simulink model "engv2_Simscape_test_no_graphs"  (R2016a)
settings: Solver=ode23t  StartTime=0.0  StopTime=5790*3  MaxStep=0.1  RelTol=1e-6
libraries: fl_lib x26, nesl_utility x23, elec_lib x8, simulink x3
settings Model: Creator=Bruno  LastModifiedBy=Bruno
settings SolverCC: MaxConsecutiveZCs=10000  ZeroCrossAlgorithm=Adaptive  AlgebraicLoopSolver=LineSearch  SolverResetMethod=Robust

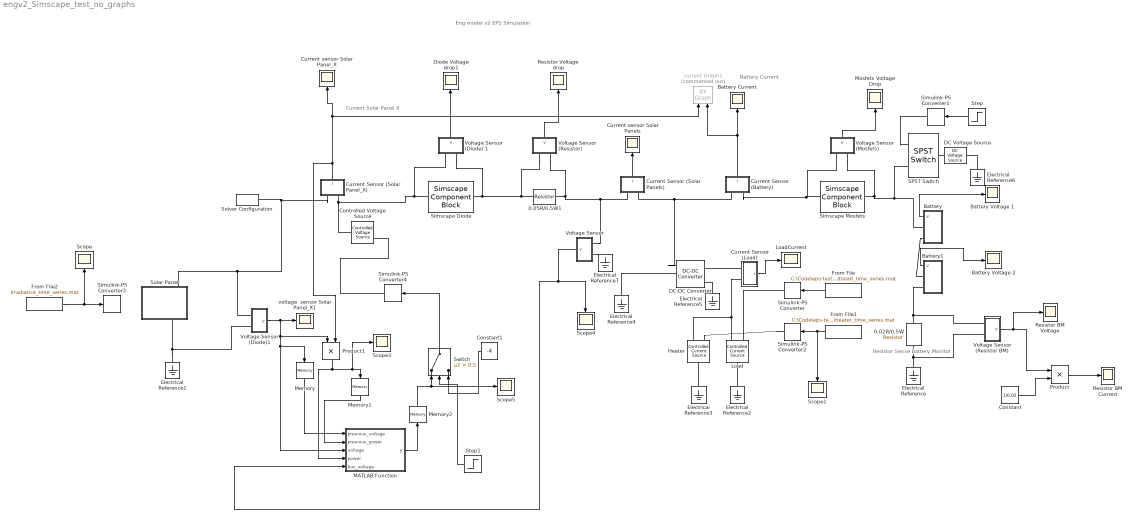
== system engv2_Simscape_test_no_graphs ==
  note: Battery Current
  note: Resistor Sense
      | Battery Monitor
  note: Current Solar Panel X
  note: Eng model v2 EPS Simulation
  " Battery" : Subsystem
      settings: CopyFcn=set_param(gcb,'LinkStatus','none')
  " Battery1" : Subsystem
      settings: CopyFcn=set_param(gcb,'LinkStatus','none')
  " 0.02R/0.5W" : elec_lib/Passive Devices/Resistor  R=0.02 Ohm  R_tol=0.01  enable_R_tol=0  tol_distribution=1  nSigma=4  enable_operating_limits=0  operating_limit_action=2  max_working_voltage=100 V  power_rating=1 W  enable_faults=0  fault_action=1  R_faulted=Inf Ohm  enable_temporal_fault=0  t_fault=1 s  enable_behavioral_fault=0  max_permissible_current=1 A  t_fail_on_current=1 s  noise_mode=0  sample_time=0.001 s  repeatability=1  auto_seed=1471942077  user_seed=0  Tdevice=25 degC  alpha=0.00393 1/K  Tmeas=25 degC  thermal_mass=100 J/K  initial_temperature=25 degC  power_derating_T1=70 degC  power_derating_T2=155 degC  operating_temperature_range_vec=[ -50 150 ] degC
  " 0.05R/0.5W1" : elec_lib/Passive Devices/Resistor  R=0.02 Ohm  R_tol=0.01  enable_R_tol=0  tol_distribution=1  nSigma=4  enable_operating_limits=0  operating_limit_action=2  max_working_voltage=100 V  power_rating=1 W  enable_faults=0  fault_action=1  R_faulted=Inf Ohm  enable_temporal_fault=0  t_fault=1 s  enable_behavioral_fault=0  max_permissible_current=1 A  t_fail_on_current=1 s  noise_mode=0  sample_time=0.001 s  repeatability=1  auto_seed=698412085  user_seed=0  Tdevice=25 degC  alpha=0.00393 1/K  Tmeas=25 degC  thermal_mass=100 J/K  initial_temperature=25 degC  power_derating_T1=70 degC  power_derating_T2=155 degC  operating_temperature_range_vec=[ -50 150 ] degC
  " Current sensor Solar Panel_X" : Scope
  " Current sensor Solar Panels" : Scope
  " Diode Voltage drop1" : Scope
  " Resistor Voltage drop" : Scope
  Battery Current : Scope
  Battery Voltage 1 : Scope
  Battery Voltage 2 : Scope
  Constant : Constant  Value=1/0.02
  Constant1 : Constant  Value=-4
  Controlled Voltage Source : fl_lib/Electrical/Electrical Sources/Controlled Voltage Source
  Current Sensor (Battery) : Subsystem
      settings: CopyFcn=set_param(gcb,'LinkStatus','none')
  Current Sensor (Load) : Subsystem
      settings: CopyFcn=set_param(gcb,'LinkStatus','none')
  Current Sensor (Solar Panel_X) : Subsystem
      settings: CopyFcn=set_param(gcb,'LinkStatus','none')
  Current Sensor (Solar Panels) : Subsystem
      settings: CopyFcn=set_param(gcb,'LinkStatus','none')
  DC Voltage Source : fl_lib/Electrical/Electrical Sources/DC Voltage Source  v0=8.4 V
  DC-DC Converter : elec_lib/Sources/DC-DC Converter  v_ref=5 V  P_rated=10 W  droop_param=1  droop=0.0 V/A  droop_percent=2  reversible=0  efficiency=99.9999  P_fixed=0.0001 mW  model_dynamics=0  tau=0.02 s  v_ini=10 V  i1_max=10 A  fault_condition=1  fault_threshold=0.5  R_fixed=100 Ohm  R_out=0.1 Ohm  fault_sign=1
  Electrical Reference{,1..7} (8 alike) : fl_lib/Electrical/Electrical Elements/Electrical Reference
  From File : FromFile  FileName=C:\Code\eps-tests\Load\load_time_series.mat
  From File1 : FromFile  FileName=C:\Code\eps-tests\Load\heater_time_series.mat
  From File2 : FromFile  FileName=irradiance_time_series.mat
  Heater : fl_lib/Electrical/Electrical Sources/Controlled Current Source
  Load : fl_lib/Electrical/Electrical Sources/Controlled Current Source
  LoadCurrent : Scope
  MATLAB Function : MATLAB Function  TreatAsAtomicUnit=on  SystemSampleTime=0.1
      settings: MinAlgLoopOccurrences=on
  Memory : Memory  X0=2.363
  Memory1 : Memory  X0=0.311*2.363
  Memory2 : Memory  X0=0.311*2.363
  Mosfets Voltage Drop : Scope
  Product : Product
  "Product1 " : Product
  Resistor BM Current : Scope
  Resistor BM Voltage : Scope
  SPST Switch : elec_lib/Passive Devices/Switches/SPST Switch  R_closed=0.01 Ohm  G_open=1e-6 S  Threshold=0 V  Width=0 V  model_dynamics=0  t_on=0.001 s  t_off=0.001 s  initial_vT=0 V
  Scope{,1,3..5} (5 alike) : Scope
  Simscape Diode : SimscapeComponentBlock  SourceFile=diode_EPS  ComponentPath=diode_EPS  ComponentVariants=diode_EPS  ComponentVariantNames=diode_EPS  ClassName=diode_EPS  SchemaVersion=1  Vt=1.38e-23 * 298 / 1.60e-19 V  R=0.0084 Ohm  n=1.00404  Is=1.3032e-6 A  i_specify=off  i_priority=None  i=1 A  v_specify=off  v_priority=None  v=0 V
      settings: CopyFcn=simscape.engine.sli.internal.componentblockcallback(gcbh,'COPY')  PreCopyFcn=simscape.engine.sli.internal.componentblockcallback(gcbh,'PRECOPY')  PreDeleteFcn=simscape.engine.sli.internal.componentblockcallback(gcbh,'PREDELETE')
      mask Type: Code produced by Embedded Systems Group - UFSC
      mask Display:
      | disp('Simscape\n\n\n')
      | disp('\n\n\ndiode_EPS');
      | color('red');
      | port_label('RConn', 1,'-');
      | port_label('LConn', 1,'+');
  "Simscape Mosfets " : SimscapeComponentBlock  SourceFile=MOSFETs_EPS  ComponentPath=MOSFETs_EPS  ComponentVariants=MOSFETs_EPS  ComponentVariantNames=MOSFETs_EPS  ClassName=MOSFETs_EPS  SchemaVersion=1  Vt=1.38e-23 * 298 / 1.60e-19 V  Rsd=0.27 Ohm  Rs=0.008235 Ohm  n=1.89492  Is=1.26064e-7 A  i_specify=off  i_priority=None  i=1 A  v_specify=off  v_priority=None  v=2 V  Vr_DC_specify=off  Vr_DC_priority=None  Vr_DC=0 V  Vr_CC_specify=off  Vr_CC_priority=None  Vr_CC=0 V
      settings: CopyFcn=simscape.engine.sli.internal.componentblockcallback(gcbh,'COPY')  PreCopyFcn=simscape.engine.sli.internal.componentblockcallback(gcbh,'PRECOPY')  PreDeleteFcn=simscape.engine.sli.internal.componentblockcallback(gcbh,'PREDELETE')
      mask Type: Code produced by Embedded Systems Group - UFSC
      mask Display:
      | disp('Simscape\n\n\n')
      | disp('\n\n\nMOSFETs_EPS');
      | color('red');
      | port_label('RConn', 1,'-');
      | port_label('LConn', 1,'+');
  Simulink-PS Converter{,1..4} (5 alike) : nesl_utility/Simulink-PS Converter  PhysicalDomain=network_engine_domain  SubClassName=ps_input  LeftPortType=input  RightPortType=output  PseudoPeriodic=off  Frequencies=[]  NoiseDistribution=none  NoiseParameters=[]  Unit=1  AffineConversion=off  InputFiltering=off  SimscapeFilterOrder=1  InputFilterTimeConstant=0.001  UdotUserProvided=1
  Solar Panel : Subsystem
      settings: CopyFcn=set_param(gcb,'LinkStatus','none')
  Solver Configuration : nesl_utility/Solver Configuration  PhysicalDomain=network_engine_domain  SubClassName=solver  LeftPortType=input  RightPortType=generic  Accelerate=off  Tones=[]  Harmonics=[]  SimulateNoise=off  Profile=off  UseLocalSampling=off  EnableSwitchedLinearOptims=on  FrequencyDomain=off  UseCCode=off  RelTol=0.001  AbsTol=1e-06  MinStep=1e-09  ToWorkspace=off  RevertToSquareIcSolve=off  NumHomotopyIterations=100  PhasorMode=off  PhasorModeNumHarmonics=1  OverrideAbsTol=off  DoDC=off  ResidualTolerance=1e-6  UseLocalSolver=off  LocalSolverChoice=NE_BACKWARD_EULER_ADVANCER  LocalSolverSampleTime=.001  DoFixedCost=off  MaxNonlinIter=3  MaxModeIter=2  LinearAlgebra=Sparse  DelaysMemoryBudget=1024  AutomaticFiltering=on  FilteringTimeConstant=0.001
  Step : Step  Before=1  After=0  SampleTime=0
  Step1 : Step  SampleTime=0
  Switch : Switch  Criteria=u2 > Threshold  Threshold=0.5
  Voltage Sensor : Subsystem
      settings: CopyFcn=set_param(gcb,'LinkStatus','none')
  Voltage Sensor (Diode) 1 : Subsystem
      settings: CopyFcn=set_param(gcb,'LinkStatus','none')
  Voltage Sensor (Diode)1 : Subsystem
      settings: CopyFcn=set_param(gcb,'LinkStatus','none')
  Voltage Sensor (Mosfets) : Subsystem
      settings: CopyFcn=set_param(gcb,'LinkStatus','none')
  Voltage Sensor (Resistor BM) : Subsystem
      settings: CopyFcn=set_param(gcb,'LinkStatus','none')
  "Voltage Sensor (Resistor) " : Subsystem
      settings: CopyFcn=set_param(gcb,'LinkStatus','none')
  current Graph1 : simulink/Sinks/XY Graph  Commented=on  xmin=-2  xmax=2  ymin=-2  ymax=2  st=-1
  voltage  sensor Solar Panel_X1 : Scope
  wires:
  Voltage Sensor (Mosfets)/1(v) -> Mosfets Voltage Drop/1
  " Battery"/1(v) -> Battery Voltage 1/1
  Current Sensor (Solar Panels)/1(i) -> " Current sensor Solar Panels"/1
  "Voltage Sensor (Resistor) "/1(v) -> " Resistor Voltage drop"/1
  Voltage Sensor (Resistor BM)/1(v) -> Product/1, Resistor BM Voltage/1
  Current Sensor (Battery)/1(i) -> current Graph1/2, Battery Current/1
  Current Sensor (Solar Panel_X)/1(i) -> "Product1 "/2, current Graph1/1, " Current sensor Solar Panel_X"/1
  Step/1 -> Simulink-PS Converter1/1
  Current Sensor (Load)/1(i) -> LoadCurrent/1
  From File/1 -> Simulink-PS Converter/1
  From File1/1 -> Scope1/1, Simulink-PS Converter2/1
  From File2/1 -> Scope/1, Simulink-PS Converter3/1
  Constant/1 -> Product/2
  Product/1 -> Resistor BM Current/1
  " Battery1"/1(v) -> Battery Voltage 2/1
  Voltage Sensor (Diode)1/1(v) -> "Product1 "/1, Memory/1, MATLAB Function/3(voltage), voltage  sensor Solar Panel_X1/1
  Memory/1 -> MATLAB Function/1(previous_voltage)
  Memory1/1 -> MATLAB Function/2(previous_power)
  "Product1 "/1 -> Scope3/1, Memory1/1, MATLAB Function/4(power)
  MATLAB Function/1(y) -> Memory2/1
  Memory2/1 -> Switch/1, Scope5/1
  Voltage Sensor/1(v) -> Scope4/1, MATLAB Function/5(bus_voltage)
  Switch/1 -> Simulink-PS Converter4/1
  Step1/1 -> Switch/2
  Constant1/1 -> Switch/3
  Voltage Sensor (Diode) 1/1(v) -> " Diode Voltage drop1"/1
  connections:
  Voltage Sensor (Resistor BM)/LConn1 -- " Battery1"/RConn2 -- " 0.02R/0.5W"/LConn1
  "Voltage Sensor (Resistor) "/LConn1 -- Voltage Sensor (Diode) 1/LConn2 -- Simscape Diode/RConn1 -- " 0.05R/0.5W1"/LConn1
  Solver Configuration/RConn1 -- Current Sensor (Solar Panel_X)/LConn1 -- Voltage Sensor (Diode)1/LConn1
  Current Sensor (Battery)/LConn1 -- DC-DC Converter/LConn1 -- Current Sensor (Solar Panels)/LConn2
  " 0.02R/0.5W"/RConn1 -- Electrical Reference/LConn1 -- Voltage Sensor (Resistor BM)/LConn2
  Current Sensor (Battery)/LConn2 -- "Simscape Mosfets "/LConn1 -- Voltage Sensor (Mosfets)/LConn1
  Electrical Reference1/LConn1 -- Voltage Sensor (Diode)1/LConn2
  Electrical Reference2/LConn1 -- Load/LConn1
  Current Sensor (Load)/LConn2 -- Heater/RConn2 -- Load/RConn2
  Electrical Reference4/LConn1 -- DC-DC Converter/LConn2
  DC-DC Converter/RConn2 -- Electrical Reference5/LConn1
  Simulink-PS Converter1/RConn1 -- SPST Switch/LConn1
  Simulink-PS Converter/RConn1 -- Load/RConn1
  Electrical Reference6/LConn1 -- DC Voltage Source/RConn1
  Current Sensor (Load)/LConn1 -- DC-DC Converter/RConn1
  DC Voltage Source/LConn1 -- SPST Switch/RConn1
  Electrical Reference3/LConn1 -- Heater/LConn1
  Simulink-PS Converter2/RConn1 -- Heater/RConn1
  " Battery1"/RConn1 -- " Battery"/RConn2
  Voltage Sensor/LConn2 -- Electrical Reference7/LConn1
  Simulink-PS Converter4/RConn1 -- Controlled Voltage Source/RConn1
  Controlled Voltage Source/LConn1 -- Voltage Sensor (Diode) 1/LConn1 -- Simscape Diode/LConn1 -- Current Sensor (Solar Panel_X)/LConn2
  Voltage Sensor/LConn1 -- " 0.05R/0.5W1"/RConn1 -- "Voltage Sensor (Resistor) "/LConn2 -- Current Sensor (Solar Panels)/LConn1
  SPST Switch/LConn2 -- "Simscape Mosfets "/RConn1 -- Voltage Sensor (Mosfets)/LConn2 -- " Battery"/RConn1

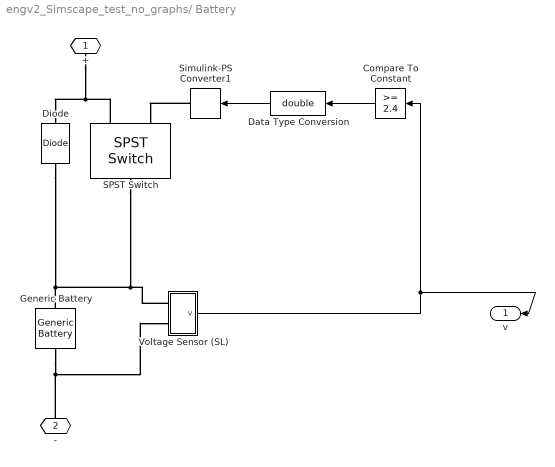
== system engv2_Simscape_test_no_graphs/ Battery ==
  Compare To Constant : simulink/Logic and Bit Operations/Compare To Constant  relop=>=  const=2.4  OutDataTypeStr=boolean
  Data Type Conversion : DataTypeConversion  OutDataTypeStr=double
  Diode : fl_lib/Electrical/Electrical Elements/Diode  Vf=0.0001 V  Ron=0.0001 Ohm  Goff=1e-8 1/Ohm  i_specify=off  i_priority=None  i=0 A  v_specify=off  v_priority=None  v=0 V
  Generic Battery : elec_lib/Sources/Generic Battery  Vnom=4.1 V  R1=0.01 Ohm  prm_AH=2  AH=3 hr*A  AH0=3 hr*A  V1=3.789 V  AH1=2.19 hr*A  prm_R2=1  R2=2e+3 Ohm
  SPST Switch : elec_lib/Passive Devices/Switches/SPST Switch  R_closed=0.01 Ohm  G_open=1e-6 S  Threshold=0 V  Width=0.1 V  model_dynamics=0  t_on=0.001 s  t_off=0.001 s  initial_vT=0 V
  Simulink-PS Converter1 : nesl_utility/Simulink-PS Converter  PhysicalDomain=network_engine_domain  SubClassName=ps_input  LeftPortType=input  RightPortType=output  PseudoPeriodic=off  Frequencies=[]  NoiseDistribution=none  NoiseParameters=[]  Unit=V  AffineConversion=off  InputFiltering=off  SimscapeFilterOrder=1  InputFilterTimeConstant=.001  UdotUserProvided=1
  Voltage Sensor (SL) : Subsystem
      settings: CopyFcn=set_param(gcb,'LinkStatus','none')
  + : PMIOPort  Port=1  Side=Right
  - : PMIOPort  Port=2  Side=Right
  v : Outport
  wires:
  Voltage Sensor (SL)/1(v) -> v/1, Compare To Constant/1
  Data Type Conversion/1 -> Simulink-PS Converter1/1
  Compare To Constant/1 -> Data Type Conversion/1
  connections:
  -/RConn1 -- Generic Battery/RConn1 -- Voltage Sensor (SL)/LConn2
  Voltage Sensor (SL)/LConn1 -- SPST Switch/RConn1 -- Diode/RConn1 -- Generic Battery/LConn1
  +/RConn1 -- Diode/LConn1 -- SPST Switch/LConn2
  Simulink-PS Converter1/RConn1 -- SPST Switch/LConn1

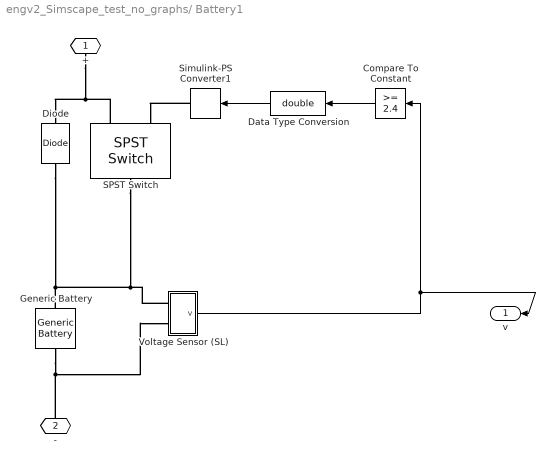
== system engv2_Simscape_test_no_graphs/ Battery1 ==
  Compare To Constant : simulink/Logic and Bit Operations/Compare To Constant  relop=>=  const=2.4  OutDataTypeStr=boolean
  Data Type Conversion : DataTypeConversion  OutDataTypeStr=double
  Diode : fl_lib/Electrical/Electrical Elements/Diode  Vf=0.0001 V  Ron=0.0001 Ohm  Goff=1e-8 1/Ohm  i_specify=off  i_priority=None  i=0 A  v_specify=off  v_priority=None  v=0 V
  Generic Battery : elec_lib/Sources/Generic Battery  Vnom=4.1 V  R1=0.01 Ohm  prm_AH=2  AH=3 hr*A  AH0=3 hr*A  V1=3.789 V  AH1=2.19 hr*A  prm_R2=1  R2=2e+3 Ohm
  SPST Switch : elec_lib/Passive Devices/Switches/SPST Switch  R_closed=0.01 Ohm  G_open=1e-6 S  Threshold=0 V  Width=0.1 V  model_dynamics=0  t_on=0.001 s  t_off=0.001 s  initial_vT=0 V
  Simulink-PS Converter1 : nesl_utility/Simulink-PS Converter  PhysicalDomain=network_engine_domain  SubClassName=ps_input  LeftPortType=input  RightPortType=output  PseudoPeriodic=off  Frequencies=[]  NoiseDistribution=none  NoiseParameters=[]  Unit=V  AffineConversion=off  InputFiltering=off  SimscapeFilterOrder=1  InputFilterTimeConstant=.001  UdotUserProvided=1
  Voltage Sensor (SL) : Subsystem
      settings: CopyFcn=set_param(gcb,'LinkStatus','none')
  + : PMIOPort  Port=1  Side=Right
  - : PMIOPort  Port=2  Side=Right
  v : Outport
  wires:
  Voltage Sensor (SL)/1(v) -> v/1, Compare To Constant/1
  Data Type Conversion/1 -> Simulink-PS Converter1/1
  Compare To Constant/1 -> Data Type Conversion/1
  connections:
  -/RConn1 -- Generic Battery/RConn1 -- Voltage Sensor (SL)/LConn2
  Voltage Sensor (SL)/LConn1 -- SPST Switch/RConn1 -- Diode/RConn1 -- Generic Battery/LConn1
  +/RConn1 -- Diode/LConn1 -- SPST Switch/LConn2
  Simulink-PS Converter1/RConn1 -- SPST Switch/LConn1

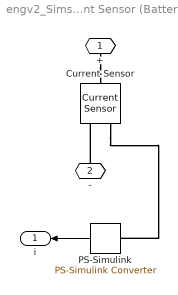
== system engv2_Simscape_test_no_graphs/Current Sensor (Battery) ==
  Current Sensor : fl_lib/Electrical/Electrical Sensors/Current Sensor
  PS-Simulink : nesl_utility/PS-Simulink Converter  PhysicalDomain=network_engine_domain  SubClassName=ps_output  LeftPortType=input  RightPortType=output  PseudoPeriodic=off  Frequencies=[]  Unit=A  AffineConversion=off
  + : PMIOPort  Port=1  Side=Left
  - : PMIOPort  Port=2  Side=Left
  i : Outport
  wires:
  PS-Simulink/1 -> i/1
  connections:
  -/RConn1 -- Current Sensor/RConn2
  +/RConn1 -- Current Sensor/LConn1
  Current Sensor/RConn1 -- PS-Simulink/LConn1

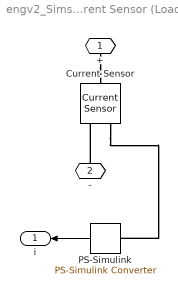
== system engv2_Simscape_test_no_graphs/Current Sensor (Load) ==
  Current Sensor : fl_lib/Electrical/Electrical Sensors/Current Sensor
  PS-Simulink : nesl_utility/PS-Simulink Converter  PhysicalDomain=network_engine_domain  SubClassName=ps_output  LeftPortType=input  RightPortType=output  PseudoPeriodic=off  Frequencies=[]  Unit=A  AffineConversion=off
  + : PMIOPort  Port=1  Side=Left
  - : PMIOPort  Port=2  Side=Left
  i : Outport
  wires:
  PS-Simulink/1 -> i/1
  connections:
  -/RConn1 -- Current Sensor/RConn2
  +/RConn1 -- Current Sensor/LConn1
  Current Sensor/RConn1 -- PS-Simulink/LConn1

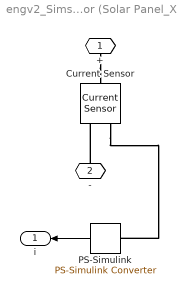
== system engv2_Simscape_test_no_graphs/Current Sensor (Solar Panel_X) ==
  Current Sensor : fl_lib/Electrical/Electrical Sensors/Current Sensor
  PS-Simulink : nesl_utility/PS-Simulink Converter  PhysicalDomain=network_engine_domain  SubClassName=ps_output  LeftPortType=input  RightPortType=output  PseudoPeriodic=off  Frequencies=[]  Unit=A  AffineConversion=off
  + : PMIOPort  Port=1  Side=Left
  - : PMIOPort  Port=2  Side=Left
  i : Outport
  wires:
  PS-Simulink/1 -> i/1
  connections:
  -/RConn1 -- Current Sensor/RConn2
  +/RConn1 -- Current Sensor/LConn1
  Current Sensor/RConn1 -- PS-Simulink/LConn1

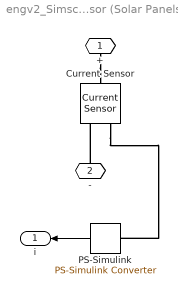
== system engv2_Simscape_test_no_graphs/Current Sensor (Solar Panels) ==
  Current Sensor : fl_lib/Electrical/Electrical Sensors/Current Sensor
  PS-Simulink : nesl_utility/PS-Simulink Converter  PhysicalDomain=network_engine_domain  SubClassName=ps_output  LeftPortType=input  RightPortType=output  PseudoPeriodic=off  Frequencies=[]  Unit=A  AffineConversion=off
  + : PMIOPort  Port=1  Side=Left
  - : PMIOPort  Port=2  Side=Left
  i : Outport
  wires:
  PS-Simulink/1 -> i/1
  connections:
  -/RConn1 -- Current Sensor/RConn2
  +/RConn1 -- Current Sensor/LConn1
  Current Sensor/RConn1 -- PS-Simulink/LConn1

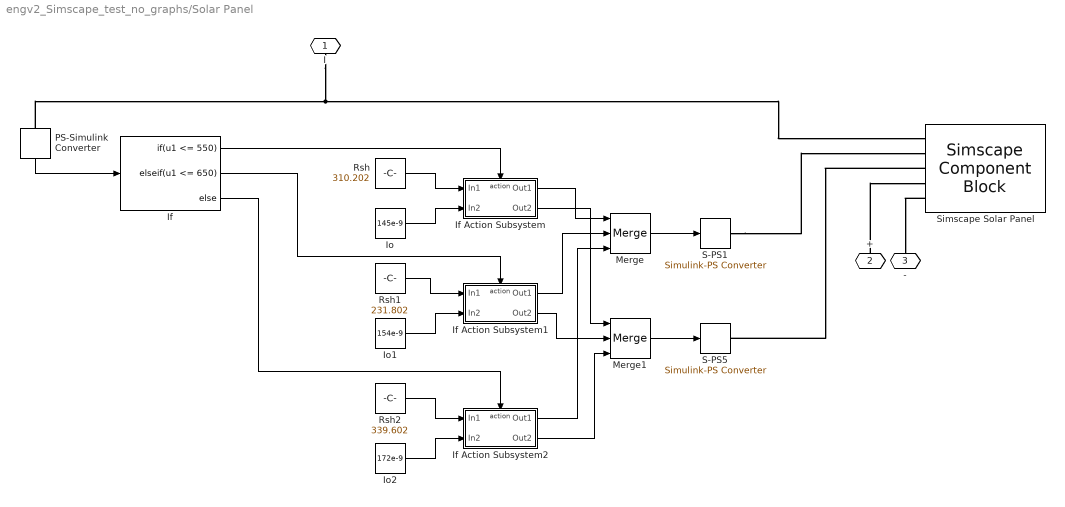
== system engv2_Simscape_test_no_graphs/Solar Panel ==
  If : If  IfExpression=u1 <= 550  ElseIfExpressions=u1 <= 650
  If Action Subsystem : Subsystem  TreatAsAtomicUnit=on
  If Action Subsystem1 : Subsystem  TreatAsAtomicUnit=on
  If Action Subsystem2 : Subsystem  TreatAsAtomicUnit=on
  Io : Constant  Value=145e-9
  Io1 : Constant  Value=154e-9
  Io2 : Constant  Value=172e-9
  Merge : Merge  Inputs=3
  Merge1 : Merge  Inputs=3
  PS-Simulink Converter : nesl_utility/PS-Simulink Converter  PhysicalDomain=network_engine_domain  SubClassName=ps_output  LeftPortType=input  RightPortType=output  PseudoPeriodic=off  Frequencies=[]  Unit=1  AffineConversion=off
  Rsh : Constant  Value=310.202
  Rsh1 : Constant  Value=231.802
  Rsh2 : Constant  Value=339.602
  S-PS1 : nesl_utility/Simulink-PS Converter  PhysicalDomain=network_engine_domain  SubClassName=ps_input  LeftPortType=input  RightPortType=output  PseudoPeriodic=off  Frequencies=[]  NoiseDistribution=none  NoiseParameters=[]  Unit=1  AffineConversion=off  InputFiltering=off  SimscapeFilterOrder=1  InputFilterTimeConstant=0.001  UdotUserProvided=1
  S-PS5 : nesl_utility/Simulink-PS Converter  PhysicalDomain=network_engine_domain  SubClassName=ps_input  LeftPortType=input  RightPortType=output  PseudoPeriodic=off  Frequencies=[]  NoiseDistribution=none  NoiseParameters=[]  Unit=1  AffineConversion=off  InputFiltering=off  SimscapeFilterOrder=1  InputFilterTimeConstant=0.001  UdotUserProvided=1
  Simscape Solar Panel : SimscapeComponentBlock  SourceFile=simscape.solarPanel  ComponentPath=simscape.solarPanel  ComponentVariants=simscape.solarPanel  ComponentVariantNames=solarPanel  ClassName=solarPanel  SchemaVersion=1  Rs=5.59404 Ohm  A=2.1  Iph0=0.050 A  Np=4  Ns=10  Npp=3  i_specify=off  i_priority=None  i=0 A  v_specify=off  v_priority=None  v=0 V
      settings: CopyFcn=simscape.engine.sli.internal.componentblockcallback(gcbh,'COPY')  PreCopyFcn=simscape.engine.sli.internal.componentblockcallback(gcbh,'PRECOPY')  PreDeleteFcn=simscape.engine.sli.internal.componentblockcallback(gcbh,'PREDELETE')
      mask Type: solarPanel
      mask Display:
      | disp('Simscape\n\n\n')
      | disp('\n\n\nsolarPanel');
      | color('red');
      | port_label('LConn', 5,'n');
      | port_label('LConn', 4,'p');
      | port_label('LConn', 3,'diode saturation current');
      | port_label('LConn', 2,'parallel resistance');
      | port_label('LConn', 1,'I');
  I : PMIOPort  Port=1  Side=Right
  + : PMIOPort  Port=2  Side=Left
  - : PMIOPort  Port=3  Side=Left
  wires:
  PS-Simulink Converter/1 -> If/1
  If/1 -> If Action Subsystem/Action
  Rsh/1 -> If Action Subsystem/1(In1)
  Io/1 -> If Action Subsystem/2(In2)
  If/2 -> If Action Subsystem1/Action
  Io1/1 -> If Action Subsystem1/2(In2)
  Rsh1/1 -> If Action Subsystem1/1(In1)
  If Action Subsystem1/1(Out1) -> Merge/2
  If Action Subsystem/1(Out1) -> Merge/1
  Merge/1 -> S-PS1/1
  If/3 -> If Action Subsystem2/Action
  Rsh2/1 -> If Action Subsystem2/1(In1)
  Io2/1 -> If Action Subsystem2/2(In2)
  If Action Subsystem2/1(Out1) -> Merge/3
  If Action Subsystem/2(Out2) -> Merge1/1
  If Action Subsystem1/2(Out2) -> Merge1/2
  If Action Subsystem2/2(Out2) -> Merge1/3
  Merge1/1 -> S-PS5/1
  connections:
  I/RConn1 -- PS-Simulink Converter/LConn1 -- Simscape Solar Panel/LConn1
  +/RConn1 -- Simscape Solar Panel/LConn4
  Simscape Solar Panel/LConn5 -- -/RConn1
  S-PS1/RConn1 -- Simscape Solar Panel/LConn2
  Simscape Solar Panel/LConn3 -- S-PS5/RConn1

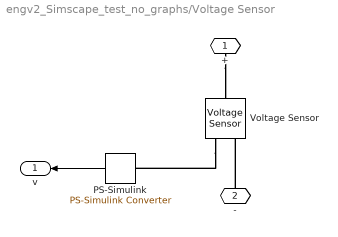
== system engv2_Simscape_test_no_graphs/Voltage Sensor ==
  PS-Simulink : nesl_utility/PS-Simulink Converter  PhysicalDomain=network_engine_domain  SubClassName=ps_output  LeftPortType=input  RightPortType=output  PseudoPeriodic=off  Frequencies=[]  Unit=V  AffineConversion=off
  Voltage Sensor : fl_lib/Electrical/Electrical Sensors/Voltage Sensor
  + : PMIOPort  Port=1  Side=Left
  - : PMIOPort  Port=2  Side=Left
  v : Outport
  wires:
  PS-Simulink/1 -> v/1
  connections:
  -/RConn1 -- Voltage Sensor/RConn2
  +/RConn1 -- Voltage Sensor/LConn1
  Voltage Sensor/RConn1 -- PS-Simulink/LConn1

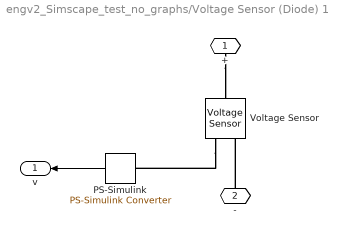
== system engv2_Simscape_test_no_graphs/Voltage Sensor (Diode) 1 ==
  PS-Simulink : nesl_utility/PS-Simulink Converter  PhysicalDomain=network_engine_domain  SubClassName=ps_output  LeftPortType=input  RightPortType=output  PseudoPeriodic=off  Frequencies=[]  Unit=V  AffineConversion=off
  Voltage Sensor : fl_lib/Electrical/Electrical Sensors/Voltage Sensor
  + : PMIOPort  Port=1  Side=Left
  - : PMIOPort  Port=2  Side=Left
  v : Outport
  wires:
  PS-Simulink/1 -> v/1
  connections:
  -/RConn1 -- Voltage Sensor/RConn2
  +/RConn1 -- Voltage Sensor/LConn1
  Voltage Sensor/RConn1 -- PS-Simulink/LConn1

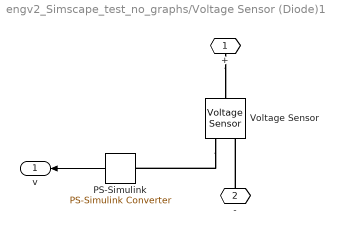
== system engv2_Simscape_test_no_graphs/Voltage Sensor (Diode)1 ==
  PS-Simulink : nesl_utility/PS-Simulink Converter  PhysicalDomain=network_engine_domain  SubClassName=ps_output  LeftPortType=input  RightPortType=output  PseudoPeriodic=off  Frequencies=[]  Unit=V  AffineConversion=off
  Voltage Sensor : fl_lib/Electrical/Electrical Sensors/Voltage Sensor
  + : PMIOPort  Port=1  Side=Left
  - : PMIOPort  Port=2  Side=Left
  v : Outport
  wires:
  PS-Simulink/1 -> v/1
  connections:
  -/RConn1 -- Voltage Sensor/RConn2
  +/RConn1 -- Voltage Sensor/LConn1
  Voltage Sensor/RConn1 -- PS-Simulink/LConn1

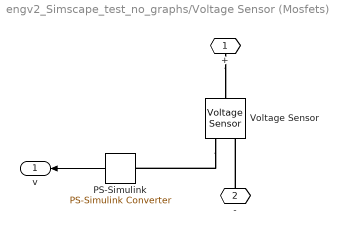
== system engv2_Simscape_test_no_graphs/Voltage Sensor (Mosfets) ==
  PS-Simulink : nesl_utility/PS-Simulink Converter  PhysicalDomain=network_engine_domain  SubClassName=ps_output  LeftPortType=input  RightPortType=output  PseudoPeriodic=off  Frequencies=[]  Unit=V  AffineConversion=off
  Voltage Sensor : fl_lib/Electrical/Electrical Sensors/Voltage Sensor
  + : PMIOPort  Port=1  Side=Left
  - : PMIOPort  Port=2  Side=Left
  v : Outport
  wires:
  PS-Simulink/1 -> v/1
  connections:
  -/RConn1 -- Voltage Sensor/RConn2
  +/RConn1 -- Voltage Sensor/LConn1
  Voltage Sensor/RConn1 -- PS-Simulink/LConn1

== system engv2_Simscape_test_no_graphs/Voltage Sensor (Resistor BM) ==
  PS-Simulink : nesl_utility/PS-Simulink Converter  PhysicalDomain=network_engine_domain  SubClassName=ps_output  LeftPortType=input  RightPortType=output  PseudoPeriodic=off  Frequencies=[]  Unit=V  AffineConversion=off
  Voltage Sensor : fl_lib/Electrical/Electrical Sensors/Voltage Sensor
  + : PMIOPort  Port=1  Side=Left
  - : PMIOPort  Port=2  Side=Left
  v : Outport
  wires:
  PS-Simulink/1 -> v/1
  connections:
  -/RConn1 -- Voltage Sensor/RConn2
  +/RConn1 -- Voltage Sensor/LConn1
  Voltage Sensor/RConn1 -- PS-Simulink/LConn1

== system engv2_Simscape_test_no_graphs/Voltage Sensor (Resistor)  ==
  PS-Simulink : nesl_utility/PS-Simulink Converter  PhysicalDomain=network_engine_domain  SubClassName=ps_output  LeftPortType=input  RightPortType=output  PseudoPeriodic=off  Frequencies=[]  Unit=V  AffineConversion=off
  Voltage Sensor : fl_lib/Electrical/Electrical Sensors/Voltage Sensor
  + : PMIOPort  Port=1  Side=Left
  - : PMIOPort  Port=2  Side=Left
  v : Outport
  wires:
  PS-Simulink/1 -> v/1
  connections:
  -/RConn1 -- Voltage Sensor/RConn2
  +/RConn1 -- Voltage Sensor/LConn1
  Voltage Sensor/RConn1 -- PS-Simulink/LConn1

== system engv2_Simscape_test_no_graphs/ Battery/Voltage Sensor (SL) ==
  PS-Simulink : nesl_utility/PS-Simulink Converter  PhysicalDomain=network_engine_domain  SubClassName=ps_output  LeftPortType=input  RightPortType=output  PseudoPeriodic=off  Frequencies=[]  Unit=V  AffineConversion=off
  Voltage Sensor : fl_lib/Electrical/Electrical Sensors/Voltage Sensor
  + : PMIOPort  Port=1  Side=Left
  - : PMIOPort  Port=2  Side=Left
  v : Outport
  wires:
  PS-Simulink/1 -> v/1
  connections:
  -/RConn1 -- Voltage Sensor/RConn2
  +/RConn1 -- Voltage Sensor/LConn1
  Voltage Sensor/RConn1 -- PS-Simulink/LConn1

== system engv2_Simscape_test_no_graphs/ Battery1/Voltage Sensor (SL) ==
  PS-Simulink : nesl_utility/PS-Simulink Converter  PhysicalDomain=network_engine_domain  SubClassName=ps_output  LeftPortType=input  RightPortType=output  PseudoPeriodic=off  Frequencies=[]  Unit=V  AffineConversion=off
  Voltage Sensor : fl_lib/Electrical/Electrical Sensors/Voltage Sensor
  + : PMIOPort  Port=1  Side=Left
  - : PMIOPort  Port=2  Side=Left
  v : Outport
  wires:
  PS-Simulink/1 -> v/1
  connections:
  -/RConn1 -- Voltage Sensor/RConn2
  +/RConn1 -- Voltage Sensor/LConn1
  Voltage Sensor/RConn1 -- PS-Simulink/LConn1

== system engv2_Simscape_test_no_graphs/Solar Panel/If Action Subsystem ==
  In1 : Inport
  In2 : Inport  Port=2
  Action Port : ActionPort  ActionType=then
  Out1 : Outport
  Out2 : Outport  Port=2
  wires:
  In1/1 -> Out1/1
  In2/1 -> Out2/1

== system engv2_Simscape_test_no_graphs/Solar Panel/If Action Subsystem1 ==
  In1 : Inport
  In2 : Inport  Port=2
  Action Port : ActionPort  ActionType=elseif
  Out1 : Outport
  Out2 : Outport  Port=2
  wires:
  In1/1 -> Out1/1
  In2/1 -> Out2/1

== system engv2_Simscape_test_no_graphs/Solar Panel/If Action Subsystem2 ==
  In1 : Inport
  In2 : Inport  Port=2
  Action Port : ActionPort  ActionType=else
  Out1 : Outport
  Out2 : Outport  Port=2
  wires:
  In1/1 -> Out1/1
  In2/1 -> Out2/1

== matlab function engv2_Simscape_test_no_graphs/MATLAB Function ==
  data: previous_voltage input; y output; previous_power input; voltage input; power input; bus_voltage input
function y = fcn(previous_voltage, previous_power, voltage, power, bus_voltage)

if power > previous_power
    if voltage > previous_voltage
        y = voltage - bus_voltage + 0.1;
    else
        y = voltage - bus_voltage - 0.1;
    end
else
    if voltage > previous_voltage
        y = voltage - bus_voltage - 0.1;
    else
        y = voltage - bus_voltage + 0.1;
    end
end

%{
if y > -2
    y = -4.2;
end
%}
